simulink model "UT-bid-cte"  (R2022a)
settings: Solver=VariableStepAuto  StartTime=0.0  StopTime=86000  RelTol=1e-3
undefined symbols (not defined in the file or in its folder): Bid_baisse, Bid_hausse, hys_max, hys_min, max_soc, min_soc, SimulationStep
libraries: Assets x3, simulink x1
settings Model: PacingRate=1000  Creator=a.dehghan  LastModifiedBy=a.dehghan

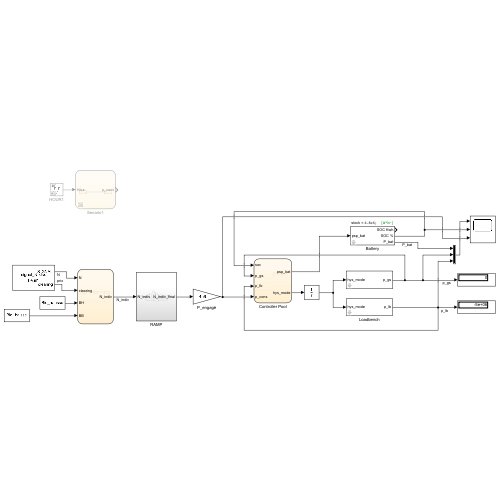
[thumbnail: Simulink's stored preview of the top-level diagram]
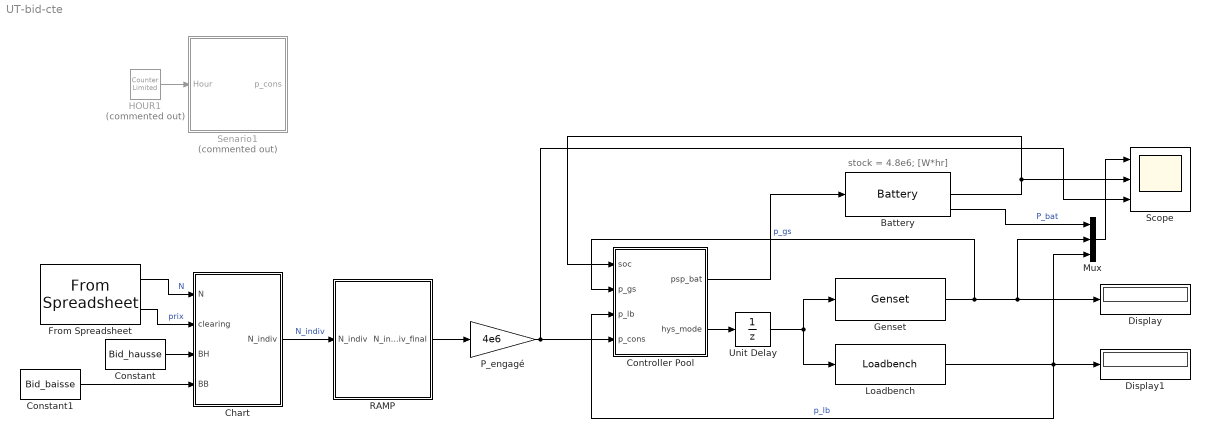
== system UT-bid-cte ==
  note: stock = 4.8e6; [W*hr]
  Battery : Assets/Battery  max_soc_limit=max_soc_limit  min_soc_limit=min_soc_limit  efficiency_discharge=efficiency_discharge  efficiency_charge=efficiency_charge  psp_bat=p  stock=stock  ini_state_of_charge=ini_state_of_charge
      settings: SourceProductName=My Library
  Chart : Stateflow chart  TreatAsAtomicUnit=on
  Constant : Constant  Value=Bid_hausse
  Constant1 : Constant  Value=Bid_baisse
  Controller Pool : Stateflow chart  TreatAsAtomicUnit=on
  Display : Display
  Display1 : Display
  From Spreadsheet : FromSpreadsheet  FileName=signal_N.xlsx  SheetName=Feuil1
  Genset : Assets/Genset  hys_mode=[0 -1]  p_max_gs=p_max_gs  rising_slew_rate=rising_slew_rate  falling_slew_rate=falling_slew_rate
      settings: SourceProductName=My Library
  HOUR1 : simulink/Sources/Counter Limited  Commented=on  uplimit=24  tsamp=3600
  Loadbench : Assets/Loadbench  hys_mode=[0 1]  p_max_lb=p_max_lb
      settings: SourceProductName=My Library
  Mux : Mux  Inputs=3
  P_engagé : Gain  Gain=4e6
  RAMP : Subsystem
  Scope : Scope  NumInputPorts=3
  Senario1 : Stateflow chart  Commented=on  TreatAsAtomicUnit=on
  Unit Delay : UnitDelay  HasFrameUpgradeWarning=on
  wires:
  Controller Pool/1(psp_bat) -> Battery/1
  Loadbench/1 -> Controller Pool/3(p_lb), Display1/1, Mux/3  "p_lb"
  Battery/3 -> Mux/1  "P_bat"
  P_engagé/1 -> Scope/3, Controller Pool/4(p_cons)
  Controller Pool/2(hys_mode) -> Unit Delay/1
  Unit Delay/1 -> Genset/1, Loadbench/1
  Battery/2 -> Scope/2, Controller Pool/1(soc)
  Genset/1 -> Controller Pool/2(p_gs), Mux/2, Display/1  "p_gs"
  HOUR1/1 -> Senario1/1(Hour)
  Chart/1(N_indiv) -> RAMP/1(N_indiv)  "N_indiv"
  Constant1/1 -> Chart/4(BB)
  Constant/1 -> Chart/3(BH)
  From Spreadsheet/1 -> Chart/1(N)  "N"
  From Spreadsheet/2 -> Chart/2(clearing)  "prix"
  RAMP/1(N_indiv_final) -> P_engagé/1
  Mux/1 -> Scope/1

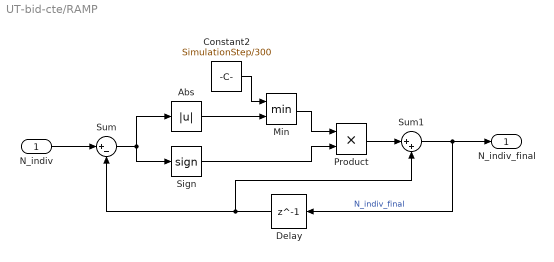
== system UT-bid-cte/RAMP ==
  N_indiv : Inport
  Abs : Abs  SaturateOnIntegerOverflow=off
  Constant2 : Constant  Value=SimulationStep/300
  Delay : Delay  DelayLength=1
  Min : MinMax  Inputs=2
  Product : Product
  Sign : Signum
  Sum : Sum  Inputs=|+-
  Sum1 : Sum  Inputs=|++
  N_indiv_final : Outport
  wires:
  Sum/1 -> Sign/1, Abs/1
  Delay/1 -> Sum/2, Sum1/2
  Product/1 -> Sum1/1
  Min/1 -> Product/1
  Sum1/1 -> Delay/1, N_indiv_final/1  "N_indiv_final"
  Sign/1 -> Product/2
  Abs/1 -> Min/2
  Constant2/1 -> Min/1
  N_indiv/1 -> Sum/1

== stateflow chart UT-bid-cte/Controller Pool ==
  state ? [commented out]
    state Battery1 [commented out]
      entry : p_cons = psp_bat;
      during :
      psp_gs = 0;
      psp_lb = 0;
    state Genset1 [commented out]
      entry : p_cons = psp_gs;
      during :
      psp_lb = 0;
      psp_bat = 0;
    state Loadbench1 [commented out]
      entry : p_cons = psp_lb
      during :
      psp_gs = 0;
      psp_bat = 0;
    ?.Battery1 -> Genset1 [commented out] : [SOC < min_soc && p_cons >=0]
    Genset1 -> ?.Battery1 [commented out] : [min_soc < SOC < max_soc]
    Genset1 -> Loadbench1 [commented out] : [SOC > max_soc && p_cons <=0]
    Loadbench1 -> Genset1 [commented out]
    Loadbench1 -> ?.Battery1 [commented out] : [min_soc < SOC < max_soc]
    ?.Battery1 -> Loadbench1 [commented out]
  state Hysteresis_mode
    state Mode___1
      en : hys_mode = -1;
      du : psp_bat = p_cons - p_lb - p_gs;
    state Mode_0
      en : hys_mode = 0;
      du : psp_bat = p_cons - p_lb - p_gs;
    state Mode_1
      en : hys_mode = 1;
      du : psp_bat = p_cons - p_lb - p_gs;
    (default) -> Mode_0
    Mode_0 -> Mode___1 [order 2] : [soc <= min_soc]
    Mode_0 -> Mode_1 [order 1] : [soc >= max_soc]
    Mode___1 -> Mode_0 : [soc >= hys_min]
    Mode_1 -> Mode_0 : [soc <= hys_max]
  state Dispatcher1 [commented out]
    state Battery1 [commented out]
      en :
      hys_mode = 0;
      p_cons = psp_bat;
    state LB_off [commented out]
      en : hys_mode = 0;
      du : p_cons = psp_bat;
    state LB_on [commented out]
      en : hys_mode = 1;
      du : p_cons = psp_lb;
    state GS_on [commented out]
      en : hys_mode = -1;
      du : p_cons = psp_gs;
    state GS_off [commented out]
      en : hys_mode = 0;
      du : p_cons = psp_bat;
    (default) -> Dispatcher1.Battery1 [commented out]
    Dispatcher1.Battery1 -> (junction 131) [commented out]
    (junction 131) -> GS_off [commented out] : [soc >= hys_min]
    (junction 131) -> LB_on [commented out] : [soc >= hys_max]
    (junction 131) -> GS_on [commented out] : [soc <= hys_min]
    (junction 131) -> LB_off [commented out] : [soc <= hys_max]
  state start_order [commented out]
    (default) -> (junction 74) [commented out] : % start_order
    (junction 74) -> (junction 75) [commented out] : [psp_gs > 0]
    (junction 74) -> (junction 76) [commented out] : {start_order = 0;}
    (junction 75) -> (junction 77) [commented out] : {start_order = 1;}
    (junction 77) -> (junction 76) [commented out]
    (junction 76) -> (junction 78) [commented out]
  state ? [commented out]
    state Battery [commented out]
      entry : p_cons = psp_bat;
      during :
      psp_gs = 0;
      psp_lb = 0;
    state Genset [commented out]
      entry : p_cons = psp_gs;
      during :
      psp_lb = 0;
      psp_bat = 0;
    state Loadbench [commented out]
      entry : p_cons = psp_lb
      during :
      psp_gs = 0;
      psp_bat = 0;
    (default) -> (junction 91) [commented out]
    (junction 91) -> Genset [commented out] : [SOC < min_soc && p_cons >=0]
    (junction 91) -> Loadbench [commented out] : [SOC > max_soc && p_cons <=0]
    (junction 91) -> Battery [commented out]
  data: soc input; p_gs input; p_lb input; psp_bat output; hys_mode output; p_cons input; min_soc parameter double; max_soc parameter double; hys_max parameter; hys_min parameter

== stateflow chart UT-bid-cte/Senario1 ==
  state decharge
    entry : p_cons = 4.5;
  state charge
    entry : p_cons = -4.5;
  (default) -> decharge
  decharge -> charge : [Hour >= 12 && Hour < 18]
  charge -> decharge : [Hour >=18]
  data: Hour input; p_cons output

== stateflow chart UT-bid-cte/Chart ==
  state Baisse
    en : clearing <= BB;
    N_indiv = -1;
  state N_0
    en : N_indiv = 0;
  state Hausse
    en :  clearing >= BH;
    N_indiv = 1;
  state Baisse1 [commented out]
    en : N_indiv = -1;
  state N_01 [commented out]
    en : N_indiv = 0;
  state Hausse1 [commented out]
    en : N_indiv = 1;
  (default) -> N_0
  Baisse -> N_0 : [N == 0]
  N_0 -> Hausse [order 1] : [N > 0 ]
  N_0 -> Baisse [order 2] : [N < 0]
  Hausse -> N_0 : [N == 0]
  (default) -> N_01 [commented out]
  Baisse1 -> N_01 [commented out] : [N == 0]
  N_01 -> Hausse1 [commented out] : [N > 0 && clearing >= BH ]
  N_01 -> Baisse1 [commented out] : [N < 0 && en : clearing <= BB ]
  Hausse1 -> N_01 [commented out] : [N == 0]
  data: N input; clearing input; BH input; BB input; N_indiv output
